simulink model "untitled1"  (R2023a)
settings: Solver=VariableStepAuto  StartTime=0.0  StopTime=10.0  RelTol=1e-3
model workspace (MAT data in the model file):
  Inertia = [0.004  0  0; 0  0.0199  0; 0  0  0.0199]
  Var = 0
settings Model: Creator=User  LastModifiedBy=User

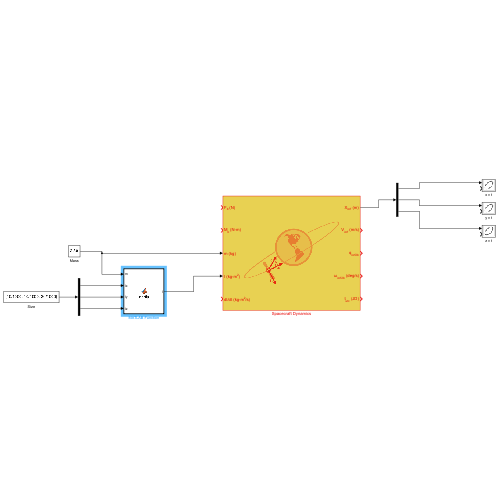
[thumbnail: Simulink's stored preview of the top-level diagram]
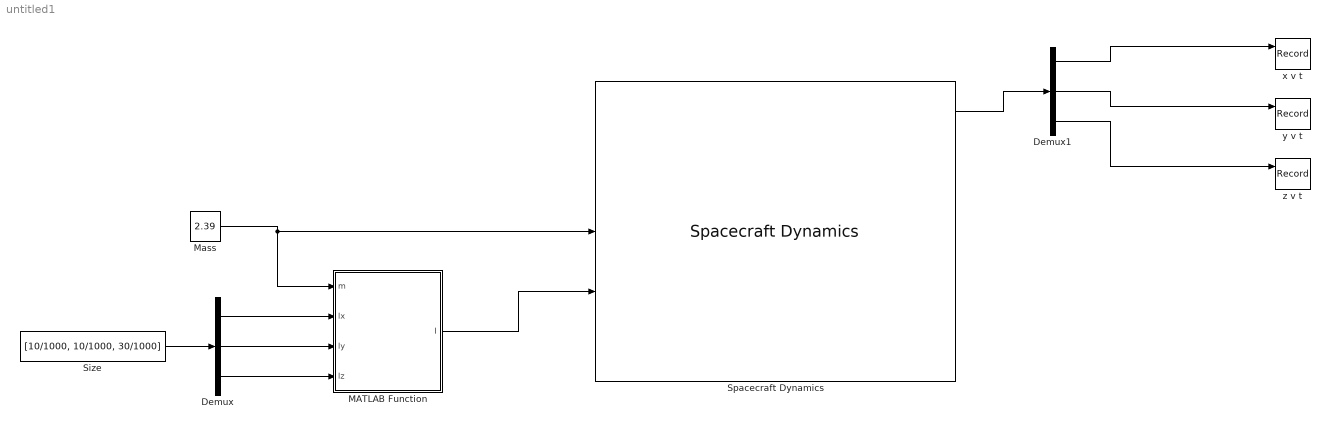
== system untitled1 ==
  Demux : Demux  Outputs=3
  Demux1 : Demux  Outputs=3
  MATLAB Function : MATLAB Function  TreatAsAtomicUnit=on
  Mass : Constant  Value=2.39
  Size : Constant  Value=[10/1000, 10/1000, 30/1000]
  Spacecraft Dynamics : SpacecraftDynamics  massType=Custom variable  mass=2.39  semiMajorAxis=(500+6378)*1000  inclination=70
  x v t : Record  FileSettingsInternal="{\"entries\":[{\"content\":{\"excelSettings\":{\"content\":{},\"type\":\"Streamout.ExcelSettings\"}},\"type\":\"Streamout.FileSettingStorage\",\"uuid\":\"9e5daaed-6cc6-4437-ac92-8e9bcf8c5133\"}],\"packageUris\":[\"http://schema.mathworks.com/mf0/streamout_blocks/R2020a\"],\"version\":\"1.0\"}"  Layout=[1 1]  SignalsInternal="{\"entries\":[{\"content\":{},\"type\":\"RecordBlkView.InputSignals\",\"uuid\":\"9f051595-3baf-4c68-b44c-e56be35e0cc2\"}],\"packageUris\":[\"http://schema.mathworks.com/mf0/streamout_blocks/R2020a\"],\"version\":\"1.0\"}"  VisualizationBindings="{\"xyplotplugin\":{\"info\":[{\"series\":[{\"bindingParametersList\":[{\"parameter\":\"X-Axis\",\"signalID\":29,\"signalName\":\"XY Graph:1\"},{\"parameter\":\"Y-Axis\",\"signalID\":32,\"signalName\":\"XY Graph:2\"}],\"seriesID\":34353}],\"subplotID\":1}]}}"  CompatibilityTag=XY
  y v t : Record  FileSettingsInternal="{\"entries\":[{\"content\":{\"excelSettings\":{\"content\":{},\"type\":\"Streamout.ExcelSettings\"}},\"type\":\"Streamout.FileSettingStorage\",\"uuid\":\"7c9e3181-36a4-47fc-a4ad-5faba19ee790\"}],\"packageUris\":[\"http://schema.mathworks.com/mf0/streamout_blocks/R2020a\"],\"version\":\"1.0\"}"  Layout=[1 1]  SignalsInternal="{\"entries\":[{\"content\":{},\"type\":\"RecordBlkView.InputSignals\",\"uuid\":\"a36c6478-1b86-4175-9df2-c861ab9ff64e\"}],\"packageUris\":[\"http://schema.mathworks.com/mf0/streamout_blocks/R2020a\"],\"version\":\"1.0\"}"  VisualizationBindings="{\"xyplotplugin\":{\"info\":[{\"series\":[{\"bindingParametersList\":[{\"parameter\":\"X-Axis\",\"signalID\":37,\"signalName\":\"XY Graph:1\"},{\"parameter\":\"Y-Axis\",\"signalID\":40,\"signalName\":\"XY Graph:2\"}],\"seriesID\":41067}],\"subplotID\":1}]}}"  CompatibilityTag=XY
  z v t : Record  FileSettingsInternal="{\"entries\":[{\"content\":{\"excelSettings\":{\"content\":{},\"type\":\"Streamout.ExcelSettings\"}},\"type\":\"Streamout.FileSettingStorage\",\"uuid\":\"a96f919d-8744-4cd3-9971-c1493379670c\"}],\"packageUris\":[\"http://schema.mathworks.com/mf0/streamout_blocks/R2020a\"],\"version\":\"1.0\"}"  Layout=[1 1]  SignalsInternal="{\"entries\":[{\"content\":{},\"type\":\"RecordBlkView.InputSignals\",\"uuid\":\"affe0916-771d-4c8f-8838-4c42d685c5cc\"}],\"packageUris\":[\"http://schema.mathworks.com/mf0/streamout_blocks/R2020a\"],\"version\":\"1.0\"}"  VisualizationBindings="{\"xyplotplugin\":{\"info\":[{\"series\":[{\"bindingParametersList\":[{\"parameter\":\"X-Axis\",\"signalID\":45,\"signalName\":\"XY Graph:1\"},{\"parameter\":\"Y-Axis\",\"signalID\":48,\"signalName\":\"XY Graph:2\"}],\"seriesID\":21921}],\"subplotID\":1}]}}"  CompatibilityTag=XY
  wires:
  Mass/1 -> Spacecraft Dynamics/3, MATLAB Function/1(m)
  Demux/2 -> MATLAB Function/3(ly)
  Demux/1 -> MATLAB Function/2(lx)
  Demux/3 -> MATLAB Function/4(lz)
  Size/1 -> Demux/1
  Spacecraft Dynamics/1 -> Demux1/1
  Demux1/1 -> x v t/1
  Demux1/2 -> y v t/1
  Demux1/3 -> z v t/1
  MATLAB Function/1(I) -> Spacecraft Dynamics/4

== matlab function untitled1/MATLAB Function ==
  data: m input; I output; lx input; ly input; lz input
function I = inertia(m, lx, ly, lz)

%%%Inertia of satellite in kg-m^2
I = (m/12)*[(lx^2+ly^2) 0 0 ;
             0 (lx^2+lz^2) 0;
             0 0 (ly^2+lz^2)];

end
